simulink model "model"  (R2021a)
settings: Solver=FixedStepDiscrete  StartTime=0.0  StopTime=1  FixedStep=1  RelTol=1e-3
undefined symbols (not defined in the file or in its folder): bias, gain
settings Model: Creator=fschwaiger  LastModifiedBy=fschwaiger
settings DataIOCC: SignalLogging=off  DSMLogging=off  SaveTime=off  ReturnWorkspaceOutputs=off

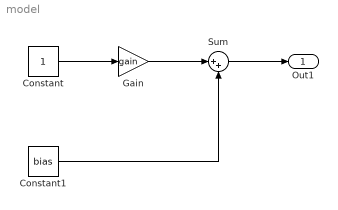
== system model ==
  Constant : Constant
  Constant1 : Constant  Value=bias
  Gain : Gain  Gain=gain
  Sum : Sum  Inputs=|++
  Out1 : Outport
  wires:
  Constant/1 -> Gain/1
  Gain/1 -> Sum/1
  Constant1/1 -> Sum/2
  Sum/1 -> Out1/1
